simulink model "M5_ScenarioReader"  (R2026a)
settings: Solver=VariableStepAuto
PreLoadFcn:
  | defineScenarioEgoPoseBus();
libraries: drivingscenarioandsensors x1
settings Model: Creator=HP  LastModifiedBy=HP

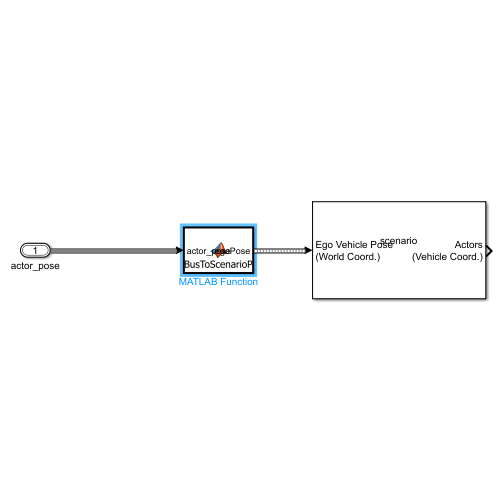
[thumbnail: Simulink's stored preview of the top-level diagram]
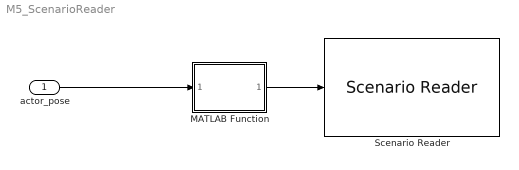
== system M5_ScenarioReader ==
  actor_pose : Inport  OutDataTypeStr=Bus: SihEgoBus
  MATLAB Function : MATLAB Function  TreatAsAtomicUnit=on
  Scenario Reader : drivingscenarioandsensors/Scenario Reader  ScenarioSource=From workspace  ScenarioFileName=EgoVehicleGoesStraight.mat  ScenarioVariableName=scenario  OutputCoordinateSystem=Vehicle coordinates  EgoVehicleSource=Input port  EgoVehicleActorID=1  OrientVehiclesOnRoad=off  OutputEgoVehiclePose=off  OutputEgoVehicleState=off  SampleTime=0.1  LaneBoundaryOutput=None  LaneBoundaryDistance=0:0.5:9.5  LaneBoundaryLocation=Center of lane markings  BusNameSource=Auto  BusName=BusActors  BusNumActorsSource=Scenario  BusNumActors=100  BusName2Source=Auto  BusName2=BusLaneBoundaries  BusNumLaneBoundariesSource=Scenario  BusNumLaneBoundaries=10  BusName3Source=Auto  BusName3=BusEgoActor  BusName4Source=Auto  BusName4=BusEgoState  ShowCoordinateLabels=on  SimulateUsing=Interpreted execution
  wires:
  MATLAB Function/1(egoPose) -> Scenario Reader/1
  actor_pose/1 -> MATLAB Function/1(actor_pose)

== matlab function M5_ScenarioReader/MATLAB Function ==
  data: actor_pose input; egoPose output Bus: ScenarioEgoPoseBus
function egoPose = egoBusToScenarioPose(actor_pose)
    egoPose.ActorID = uint32(1);
    egoPose.Position = [actor_pose.x; actor_pose.y; 0];
    egoPose.Velocity = [actor_pose.velocity; 0; 0];
    egoPose.Roll = 0;
    egoPose.Pitch = 0;
    egoPose.Yaw = actor_pose.yaw * 180/pi;
    egoPose.AngularVelocity = [0; 0; 0];
end
